simulink model "Longitudinaldynamicmodel_SmartFortwo"  (R2018b)
settings: Solver=FixedStepAuto  StartTime=0.0  StopTime=1  FixedStep=0.01  RelTol=1e-3
values from neighbouring files (symbols this model uses):
  VehMass = 988.5    [Longitudinaldynamicmodel_SmartFortwo_Parameterfile.m]
undefined symbols (not defined in the file or in its folder): DiscIntNeverNeededParam
libraries: Constant_Environment x1, Driver_PI x1, Longitudinal_DrivingCycles x1, Acceleration_Calculation x1, Air_Resistance x1, Roll_Resistance x1, Slope_Resistance x1, Constant_Power_Source x1, Simple_Auxiliary x1, Electric_Drive_Tabled_Consumption x1, Gear_Stage x1, DCAC_Converter x1
(part 2 of 3)

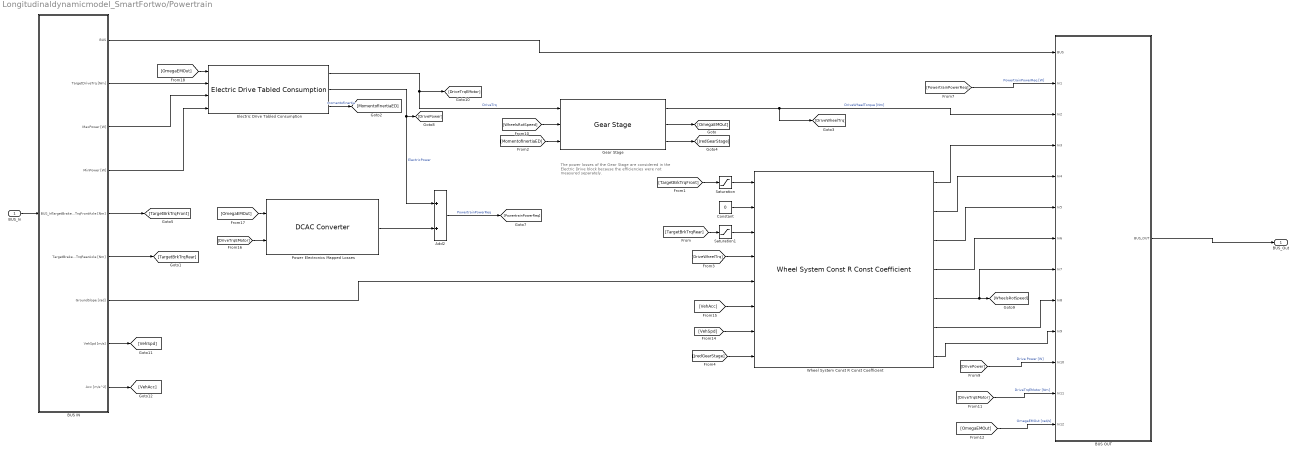
== system Longitudinaldynamicmodel_SmartFortwo/Powertrain ==
  note: The power losses of the Gear Stage are considered
      | in the Electric Drive block because the efficiencies were
      | not measured separately.
  BUS_In : Inport
  Add2 : Sum
  BUS IN : Subsystem
      mask help:
      | <Author> Alexander Koch based on Stefan Müller, Stephan Rohr
      | <Date> 02/05/2017
      |
      | <Description>
      | Automated BUS IN Block for the Bus System. After the Bus In is connected and receives signals it is possible to choose the required signals by clicking on the block. After choosing the signals it is possible to push the Refresh button. This button builds the required amount of outputs, connects the Bus Selector and the Outputs and rename all the outputs with the corresponding signal name.
      |
      | The Block automaticlly disconnects the link to the library block after opening the first time
      |
      | <Parameters>
      | -
      |
      | <Inputs>
      | Bus [Bus]
      |
      | <Outputs>
      | Bus [Bus]
      | SignalName[-]
      mask init:
      | BusInInitFct()
      settings: OpenFcn=|
      | set_param(gcb(),'LinkStatus','none')
      | open_system(gcb(),'mask')
      | open_system(strcat(gcb(),'/Bus Selector'),'Parameter')
      mask DialogControl ParameterGroupVar Prompt: Refresh
      mask DialogControl RefreshOutputs Prompt: Refresh all Output Names
      mask DialogControl RefreshOutputs Callback: BusInInitFct()
  BUS OUT : Subsystem  mask{NumberofInputs=12, NameSys='Powertrain'}
      mask prompts: NumberofInputs "Numper of costum inputs"; NameSys "Name of Bus Subsystem"
      mask help:
      | <Author> Alexander Koch based on Stefan Müller, Stephan Rohr
      | <Date> 02/05/2017
      |
      | <Description>
      | Automated BUS Out Block for the Bus System. Allows to enter the Number of costum inputs and the name of the bus system. After entering the parameters the required amout of Inputs are built and connected to the Bus Creator. The signal names that are connected to the inputs In1, ..., InN are automatically adopted at the Bus signal names and can be found in the Bus under the name of the Bus Subsystem. If the signal (line) to the Inport has no name, the name of the previous blocks outport is taken. If this is not possible, the name if the previous block is taken for the Bus signal name.
      |
      | Additional, there are two buttons. The Refresh Input Names refreshes all Input Names. This is required if signal names are changed or signals are connected for the first time. To build a new system or if another Subsystem is added between existing subsystems, the Refresh Bus Selector is required at every subsystem that is calculated after the new subsystem.
      |
      | The Block automaticlly disconnects the link to the library block after opening the first time
      |
      | <Parameters>
      | Number of costum inputs [-]
      | Name of Bus Subsystem ['abc']
      |
      | <Inputs>
      | Bus [Bus]
      | In1 [ ]
      |
      | <Outputs>
      | Bus [Bus]
      mask init:
      | BusRefreshInputs()
      settings: OpenFcn=|
      | set_param(gcb(),'LinkStatus','none')
      | open_system(gcb(),'mask')
      mask DialogControl Container3 Prompt: Refresh
      mask DialogControl RefreshInputNames Prompt: Refresh Input Names
      mask DialogControl RefreshInputNames Callback: BusRefreshLineNames()
      mask DialogControl RefreshBusSelector Prompt: Refresh Bus Selector
      mask DialogControl RefreshBusSelector Callback: BusRefreshBusSelector()
  Constant : Constant  Value=0
  Electric Drive Tabled Consumption : Electric_Drive_Tabled_Consumption/Electric Drive Tabled Consumption  inertia=0.03  mass=1  OM_M_Pel_Map=[0 84.6925537915840 106.777901162710 132.451481077187 158.717445659769 189.583562564064 219.947567848300 253.359271731562 287.719734913549 325.267898465954 364.560585120281 403.200274983864 447.563591693892 492.828790386663 540.691726349864 590.166785808662 636.561358483905 684.766906055931 734.137596997731 789.985532553104 857.853179816674 908.827398035181 961.684563108046 1019.52904110769 1081.52112973929 1143.57712046773 1200.78427519799 1267.27434692366 1330.96763225908 1399.91145341150 1460.96283186014 1522.13532912128 1591.13337312260 1654.62568484686 1718.49067047593 1783.14030989899 1852.47991946389 1921.56456923299 1990.91312442103 2061.30678608583 2131.34426123832 2203.05270027821 2289.55226312012 2376.68282420177 2454.52733777355 2530.75949498243 2607.34099640618 2684.42711031811 2763.34508226637 2845.97385304829 2963.00280011347 3052.53326845787 3134.40614789669 3225.26823505504 3314.19457665049 3406.50541394017 3500.20227762135 3591.35102796290 3685.03225906601 3782.98250894227 3881.87095410315 3980.79391338854 4076.30627526000 4181.94930220964 4286.97881720375 4389.92406519024 4497.41842284860 4603.47594352982 4710.85061726193 4818.54315585332 4930.22331092001 5041.15761416958 5166.37122862945 5276.81725954101 5387.76544736434 5521.32616802780 5637.26001511646 5761.43879713315 5886.21150930422 6012.17873781274 6142.71364240950 6280.27669163038 5676.19543942961 5258.13958693589 5295.58110214479 5435.21609088646 5171.11785981694 5274.97483494523 5470.31098908416 5158.84365253269 5768.15695867421 5696.91368959506 6048.96408164810 6479.69942526134 6479.69942526134 6479.69942526134 6479.69942526134 6479.69942526134 6479.69942526134 6479.69942526134;0 84.6925537915840 106.777901162710 132.451481077187 158.717445659769 189.583562564064 219.947567848300 253.359271731562 287.719734913549 325.267898465954 364.560585120281 403.200274983864 447.563591693892 492.828790386663 540.691726349864 590.166785808662 636.561358483905 684.766906055931 734.137596997731 789.985532553104 857.853179816674 908.827398035181 961.684563108046 1019.52904110769 1081.52112973929 1143.57712046773 1200.78427519799 1267.27434692366 1330.96763225908 1399.91145341150 1460.96283186014 1522.13532912128 1591.13337312260 1654.62568484686 1718.49067047593 1783.14030989899 1852.47991946389 1921.56456923299 1990.91312442103 2061.30678608583 2131.34426123832 2203.05270027821 2289.55226312012 2376.68282420177 2454.52733777355 2530.75949498243 2607.34099640618 2684.42711031811 2763.34508226637 2845.97385304829 2963.00280011347 3052.53326845787 3134.40614789669 3225.26823505504 3314.19457665049 3406.50541394017 3500.20227762135 3591.35102796290 3685.03225906601 3782.98250894227 3881.87095410315 3980.79391338854 4076.30627526000 4181.94930220964 4286.97881720375 4389.92406519024 4497.41842284860 4603.47594352982 4710.85061726193 4818.54315585332 4930.22331092001 5041.15761416958 5166.37122862945 5276.81725954101 5387.76544736434 5521.32616802780 5637.26001511646 5761.43879713315 5886.21150930422 6012.17873781274 6142.71364240950 6280.27669163038 5676.19543942961 5258.13958693589 5295.58110214479 5435.21609088646 5171.11785981694 5274.97483494523 5470.31098908416 5158.84365253269 5768.15695867421 5696.91368959506 6048.96408164810 6479.69942526134 6479.69942526134 6479.69942526134 6479.69942526134 6479.69942526134 6479.69942526134 6479.69942526134;0 84.6925537915840 106.777901162710 132.451481077187 158.717445659769 189.583562564064 219.947567848300 253.359271731562 287.719734913549 325.267898465954 364.560585120281 403.200274983864 447.563591693892 492.828790386663 540.691726349864 590.166785808662 636.561358483905 684.766906055931 734.137596997731 789.985532553104 857.853179816674 908.827398035181 961.684563108046 1019.52904110769 1081.52112973929 1143.57712046773 1200.78427519799 1267.27434692366 1330.96763225908 1399.91145341150 1460.96283186014 1522.13532912128 1591.13337312260 1654.62568484686 1718.49067047593 1783.14030989899 1852.47991946389 ...(+366716 chars)]  M_MotVector=[0 1.36363636363636 2.72727272727273 4.09090909090909 5.45454545454545 6.81818181818182 8.18181818181818 9.54545454545455 10.9090909090909 12.2727272727273 13.6363636363636 15.0000000000000 16.3636363636364 17.7272727272727 19.0909090909091 20.4545454545455 21.8181818181818 23.1818181818182 24.5454545454545 25.9090909090909 27.2727272727273 28.6363636363636 30.0000000000000 31.3636363636364 32.7272727272727 34.0909090909091 35.4545454545455 36.8181818181818 38.1818181818182 39.5454545454545 40.9090909090909 42.2727272727273 43.6363636363636 45 46.3636363636364 47.7272727272727 49.0909090909091 50.4545454545455 51.8181818181818 53.1818181818182 54.5454545454545 55.9090909090909 57.2727272727273 58.6363636363636 60.0000000000000 61.3636363636364 62.7272727272727 64.0909090909091 65.4545454545455 66.8181818181818 68.1818181818182 69.5454545454546 70.9090909090909 72.2727272727273 73.6363636363636 75 76.3636363636364 77.7272727272727 79.0909090909091 80.4545454545455 81.8181818181818 83.1818181818182 84.5454545454546 85.9090909090909 87.2727272727273 88.6363636363636 90 91.3636363636364 92.7272727272727 94.0909090909091 95.4545454545455 96.8181818181818 98.1818181818182 99.5454545454546 100.909090909091 102.272727272727 103.636363636364 105 106.363636363636 107.727272727273 109.090909090909 110.454545454545 111.818181818182 113.181818181818 114.545454545455 115.909090909091 117.272727272727 118.636363636364 120 121.363636363636 122.727272727273 124.090909090909 125.454545454545 126.818181818182 128.181818181818 129.545454545455 130.909090909091 132.272727272727 133.636363636364 135]  OM_MotVector=[0 3.13202920563366 6.26405841126732 9.39608761690098 12.5281168225346 15.6601460281683 18.7921752338020 21.9242044394356 25.0562336450693 28.1882628507029 31.3202920563366 34.4523212619703 37.5843504676039 40.7163796732376 43.8484088788712 46.9804380845049 50.1124672901386 53.2444964957722 56.3765257014059 59.5085549070395 62.6405841126732 65.7726133183069 68.9046425239405 72.0366717295742 75.1687009352078 78.3007301408415 81.4327593464752 84.5647885521088 87.6968177577425 90.8288469633761 93.9608761690098 97.0929053746435 100.224934580277 103.356963785911 106.488992991544 109.621022197178 112.753051402812 115.885080608445 119.017109814079 122.149139019713 125.281168225346 128.413197430980 131.545226636614 134.677255842247 137.809285047881 140.941314253515 144.073343459148 147.205372664782 150.337401870416 153.469431076049 156.601460281683 159.733489487317 162.865518692950 165.997547898584 169.129577104218 172.261606309851 175.393635515485 178.525664721119 181.657693926752 184.789723132386 187.921752338020 191.053781543653 194.185810749287 197.317839954921 200.449869160554 203.581898366188 206.713927571822 209.845956777455 212.977985983089 216.110015188723 219.242044394356 222.374073599990 225.506102805624 228.638132011257 231.770161216891 234.902190422524 238.034219628158 241.166248833792 244.298278039425 247.430307245059 250.562336450693 253.694365656326 256.826394861960 259.958424067594 263.090453273227 266.222482478861 269.354511684495 272.486540890128 275.618570095762 278.750599301396 281.882628507029 285.014657712663 288.146686918297 291.278716123930 294.410745329564 297.542774535198 300.674803740831 303.806832946465 306.938862152099 310.070891357732 313.202920563366 316.334949769000 319.466978974633 322.599008180267 325.731037385901 328.863066591534 331.995095797168 335.127125002802 338.259154208435 341.391183414069 344.523212619703 347.655241825336 350.787271030970 353.919300236604 357.051329442237 360.183358647871 363.315387853505 366.447417059138 369.579446264772 372.711475470406 375.843504676039 378.975533881673 382.107563087307 385.239592292940 388.371621498574 391.503650704208 394.635679909841 397.767709115475 400.899738321108 404.031767526742 407.163796732376 410.295825938009 413.427855143643 416.559884349277 419.691913554910 422.823942760544 425.955971966178 429.088001171811 432.220030377445 435.352059583079 438.484088788712 441.616117994346 444.748147199980 447.880176405613 451.012205611247 454.144234816881 457.276264022514 460.408293228148 463.540322433782 466.672351639415 469.804380845049 472.936410050683 476.068439256316 479.200468461950 482.332497667584 485.464526873217 488.596556078851 491.728585284485 494.860614490118 497.992643695752 501.124672901386 504.256702107019 507.388731312653 510.520760518287 513.652789723920 516.784818929554 519.916848135188 523.048877340821 526.180906546455 529.312935752089 532.444964957722 535.576994163356 538.709023368990 541.841052574623 544.973081780257 548.105110985890 551.237140191524 554.369169397158 557.501198602791 560.633227808425 563.765257014059 566.897286219692 570.029315425326 573.161344630960 576.293373836593 579.425403042227 582.557432247861 585.689461453494 588.821490659128 591.953519864762 595.085549070395 598.217578276029 601.349607481663 604.481636687296 607.613665892930 610.745695098564 613.877724304197 617.009753509831 620.141782715465 623.273811921098 626.405841126732 629.537870332366 632.669899537999 635.801928743633 638.933957949267 642.065987154900 645.198016360534 648.330045566168 651.462074771801 654.594103977435 657.726133183069 660.858162388702 663.990191594336 667.122220799970 670.254250005603 673.386279211237 676.518308416871 679.650337622504 682.782366828138 685.914396033772]  M_Full_Load=[128 128 128 127 127 126 126 126 126 124 119 114 109 103 100 94 89 85 79 75 70 68 67 65 63 62 60 58 59 60 62 63 63 62 61 60 58 57 55 53 51 50 48 46 45 43 42 40 39 38 36 35 34 32 31 30 29 28 26 25 24]  OM_Full_Load=[0 11.4144533080429 22.8289066160858 34.2433599241288 45.6578132321717 57.1769862953342 68.5914396033771 80.0058929114201 91.4203462194630 102.834799527506 114.249252835549 125.663706143592 137.078159451635 148.492612759678 160.011785822840 171.426239130883 182.840692438926 194.255145746969 205.669599055012 217.084052363055 228.498505671098 239.912958979141 251.327412287183 262.846585350346 274.261038658389 285.675491966432 297.089945274475 308.504398582518 319.918851890561 331.333305198604 342.747758506646 354.162211814689 365.681384877852 377.095838185895 388.510291493938 399.924744801981 411.339198110024 422.753651418066 434.168104726109 445.582558034152 456.997011342195 468.516184405358 479.930637713401 491.345091021444 502.759544329487 514.173997637529 525.588450945572 537.002904253615 548.417357561658 559.831810869701 571.350983932864 582.765437240907 594.179890548950 605.594343856992 617.008797165035 628.423250473078 639.837703781121 651.252157089164 662.666610397207 674.185783460370 685.600236768413]  M_Min_Load=[0 0 0 0 0 0 0 0 0 0 0 0 0 0 0 0 0 0 0 0 0 0 0 0 0 0 0 0 0 0 0 0 0 0 0 0 0 0 0 0 0 0 0 0 0 0 0 0 0 0 0 0 0 0 0 0 0 0 0 0 0]  OM_Min_Load=[0 11.4144533080429 22.8289066160858 34.2433599241288 45.6578132321717 57.1769862953342 68.5914396033771 80.0058929114201 91.4203462194630 102.834799527506 114.249252835549 125.663706143592 137.078159451635 148.492612759678 160.011785822840 171.426239130883 182.840692438926 194.255145746969 205.669599055012 217.084052363055 228.498505671098 239.912958979141 251.327412287183 262.846585350346 274.261038658389 285.675491966432 297.089945274475 308.504398582518 319.918851890561 331.333305198604 342.747758506646 354.162211814689 365.681384877852 377.095838185895 388.510291493938 399.924744801981 411.339198110024 422.753651418066 434.168104726109 445.582558034152 456.997011342195 468.516184405358 479.930637713401 491.345091021444 502.759544329487 514.173997637529 525.588450945572 537.002904253615 548.417357561658 559.831810869701 571.350983932864 582.765437240907 594.179890548950 605.594343856992 617.008797165035 628.423250473078 639.837703781121 651.252157089164 662.666610397207 674.185783460370 685.600236768413]  LocalSampleTime=-1
  Gear Stage : Gear_Stage/Gear Stage  iGear=i_gear  eta=1  JredGetr=0.19  LocalSampleTime=-1
  Power Electronics Mapped Losses : DCAC_Converter/DCAC Converter  W_Vektor=[0 10.4719755119660 21.7817090648892 33.0914426178125 44.4011761707357 55.7109097236590 67.0206432765823 78.3303768295055 89.6401103824288 100.949843935352 112.259577488275 123.569311041199 134.879044594122 146.188778147045 157.498511699968 168.808245252892 180.117978805815 191.427712358738 202.737445911661 214.047179464585 225.356913017508 236.666646570431 247.976380123354 259.286113676278 270.595847229201 281.905580782124 293.215314335047 304.525047887971 315.834781440894 327.144514993817 338.454248546740 349.763982099664 361.073715652587 372.383449205510 383.693182758433 395.002916311357 406.312649864280 417.622383417203 428.932116970126 440.241850523050 451.551584075973 462.861317628896 474.171051181819 485.480784734743 496.790518287666 508.100251840589 519.409985393512 530.719718946436 542.029452499359 553.339186052282 564.648919605206 575.958653158129 587.268386711052 598.578120263975 609.887853816898 621.197587369822 632.507320922745 643.817054475668 655.126788028592 666.436521581515 677.746255134438]  M_Vektor_motgen=[0 1 2 3 4 5 6 7 8 9 10 11 12 13 14 15 16 17 18 19 20 21 22 23 24 25 26 27 28 29 30 31 32 33 34 35 36 37 38 39 40 41 42 43 44 45 46 47 48 49 50 51 52 53 54 55 56 57 58 59 60 61 62 63 64 65 66 67 68 69 70 71 72 73 74 75 76 77 78 79 80 81 82 83 84 85 86 87 88 89 90 91 92 93 94 95 96 97 98 99 100 101 102 103 104 105 106 107 108 109 110 111 112 113 114 115 116 117 118 119 120 121 122 123 124 125 126 127 128 129 130]  P_Loss=[0 0 0 0 0 0 0 0 0 0 0 0 0 0 0 0 0 0 0 0 0 0 0 0 0 0 0 0 0 0 0 0 0 0 0 0 0 0 0 0 0 0 0 0 0 0 0 0 0 0 0 0 0 0 0 0 0 0 0 0 0 0 0 0 0 0 0 0 0 0 0 0 0 0 0 0 0 0 0 0 0 0 0 0 0 0 0 0 0 0 0 0 0 0 0 0 0 0 0 0 0 0 0 0 0 0 0 0 0 0 0 0 0 0 0 0 0 0 0 0 0 0 0 0 0 0 0 0 0 0 0;0 82 70 84 90 100 106 112 101 115 122 130 144 146 153 162 154 169 188 198 202 216 231 236 247 260 271 279 293 309 316 326 335 353 373 392 407 427 437 460 475 478 493 505 523 529 551 565 570 582 598 616 631 647 665 682 700 716 730 726 743 763 780 805 824 840 861 884 903 919 947 960 981 995 1018 1041 1062 1086 1110 1130 1152 1170 1188 1211 1237 1259 1280 1302 1323 1344 1369 1392 1412 1440 1460 1493 1518 1540 1568 1594 1617 1646 1670 1709 1743 1769 1791 1825 1856 1881 1938 2212 3001 3444 3441 3510 3626 3825 3876 3879 3957 4140 4177 3954 4094 3971 3839 3839 3839 3839 3839;0 61 78 75 74 73 81 94 94 97 96 106 120 131 139 145 154 169 180 188 198 206 215 230 242 254 265 268 286 302 306 318 344 370 384 399 410 423 438 458 483 500 512 520 528 539 554 573 589 600 614 632 645 655 678 691 714 720 739 748 763 777 787 809 833 829 860 887 913 937 949 962 976 988 1007 1032 1049 1076 1095 1118 1143 1168 1192 1212 1231 1256 1293 1323 1337 1356 1387 1406 1427 1456 1469 1496 1515 1558 1577 1607 1643 1675 1694 1710 1739 1772 1805 1832 1870 1893 1924 1942 1976 1999 2049 2640 3767 4034 4108 4084 4241 4351 4407 4486 4544 4620 3839 3839 3839 3839 3839;0 70 71 95 83 94 92 96 105 107 112 125 141 143 150 153 165 176 190 203 218 233 240 245 253 260 274 285 304 329 341 352 358 365 379 403 424 444 460 472 483 499 525 535 543 561 575 589 597 611 632 643 656 664 677 700 719 731 742 759 777 794 814 839 858 870 892 917 938 953 968 987 1008 1022 1035 1055 1085 1111 1129 1151 1176 1192 1213 1240 1276 1296 1325 1348 1369 1387 1405 1432 1465 1493 1507 1525 1558 1586 1614 1642 1663 1683 1718 1753 1777 1801 1832 1860 1893 1925 1956 1984 2007 2030 2062 2093 2124 2160 2187 2222 2252 2304 2714 4353 4916 3997 3839 3839 3839 3839 3839;0 74 50 130 190 192 101 114 128 71 125 147 164 97 157 185 186 201 216 227 232 238 241 252 264 279 293 306 320 335 355 350 365 394 396 405 423 436 452 468 481 497 508 518 532 545 554 569 588 604 613 625 645 667 677 690 709 726 745 765 780 791 803 829 843 855 881 897 912 926 942 967 994 1017 1036 1056 1073 1104 1121 1152 1181 1210 1240 1264 1282 1303 1323 1349 1371 1396 1415 1439 1469 1495 1515 1540 1563 1591 1625 1648 1677 1706 1736 1764 1793 1824 1842 1877 1912 1945 1975 2002 2024 2048 2081 2116 2143 2180 2207 2259 2278 2340 2348 2402 2412 3130 3839 3839 3839 3839 3839;0 97 63 80 77 71 70 92 102 101 123 143 135 155 167 123 148 166 185 200 226 242 265 255 265 280 315 323 318 335 346 366 381 399 417 422 439 455 469 485 498 512 525 539 550 574 587 589 608 620 642 662 668 685 705 718 725 738 758 776 792 805 834 852 859 885 897 923 947 967 985 998 1012 1023 1052 1079 1100 1125 1143 1167 1187 1214 1253 1276 1309 1333 1360 1375 1400 1424 1445 1464 1482 1504 1536 1562 1591 1615 1648 1680 1708 1734 1763 1796 1819 1825 1852 1870 1910 1946 1979 2013 2048 2088 2118 2153 2189 2216 2239 2276 2311 2337 2377 2430 2439 3130 3839 3839 3839 3839 3839;0 54 47 58 68 60 51 67 76 84 98 114 113 116 128 138 140 157 175 171 180 195 214 221 231 239 258 265 274 290 315 334 355 377 405 415 432 449 467 482 502 518 521 532 552 558 572 584 600 622 634 651 666 679 694 714 726 740 762 782 800 820 833 853 876 894 914 931 953 971 981 991 1011 1036 1068 1088 1111 1128 1142 1166 1197 1229 1255 1273 1304 1348 1379 1414 1440 1454 1475 1496 1514 1537 1564 1589 1611 1605 1652 1678 1706 1735 1768 1805 1835 1862 1903 1936 1962 2002 2036 2057 2079 2113 2149 2183 2212 2244 2285 2323 2355 2386 2410 2437 2457 3130 3839 3839 3839 3839 3839;0 78 78 96 96 93 93 106 115 120 127 134 146 157 157 161 179 196 182 188 211 212 224 245 260 287 306 309 317 325 338 356 376 399 405 416 447 470 487 494 492 494 517 534 542 561 575 584 604 625 635 656 668 681 703 723 742 765 786 804 816 829 843 864 889 904 916 929 942 962 992 1019 1036 1061 1082 ...(+31348 chars)]  LocalSampleTime=-1
  Saturation : Saturate  UpperLimit=0  LowerLimit=-inf
  Saturation1 : Saturate  UpperLimit=0  LowerLimit=-inf
  Wheel System Const R Const Coefficient : Wheel_System_Const_R/Wheel System Const R Const Coefficient  Wheel_Radius=r_dyn  Wheel_Roll_Resistance=0.0185  Wheel_Roll_Resistance_Dyn=0  mu_Tyre=0.7  J_FourWheels=4  Gravity=gravity  Wheelbase=1.863  COG_Height=0.5  COG_Front=1.1178  COG_Rear=0.7452  Veh_Mass=VehMass  LocalSampleTime=-1
  BUS_Out : Outport
  wires:
  BUS IN/1(BUS) -> BUS OUT/1(BUS)
  BUS_In/1 -> BUS IN/1(BUS_In)
  [TargetBrkTrqFront] -> Saturation/1
  [TargetBrkTrqRear] -> Saturation1/1
  BUS IN/5(TargetBrakeTrqFrontAxle [Nm]) -> [TargetBrkTrqFront]
  BUS IN/2(TargetDriveTrq [Nm]) -> Electric Drive Tabled Consumption/2
  Electric Drive Tabled Consumption/1 -> Gear Stage/1, [DriveTrqEMotor]  "DriveTrq"
  Gear Stage/2 -> [OmegaEMOut]
  Constant/1 -> Wheel System Const R Const Coefficient/2
  [MomentofInertiaED] -> Gear Stage/3
  Gear Stage/1 -> [DriveWheelTrq], BUS OUT/3(In2)  "DriveWheelTorque [Nm]"
  [DriveWheelTrq] -> Wheel System Const R Const Coefficient/4
  Gear Stage/3 -> [JredGearStage]
  [JredGearStage] -> Wheel System Const R Const Coefficient/8
  Wheel System Const R Const Coefficient/1 -> BUS OUT/4(In3)
  Wheel System Const R Const Coefficient/2 -> BUS OUT/5(In4)
  Wheel System Const R Const Coefficient/3 -> BUS OUT/6(In5)
  Wheel System Const R Const Coefficient/4 -> BUS OUT/7(In6)
  Wheel System Const R Const Coefficient/5 -> [WheelsRotSpeed], BUS OUT/8(In7)
  Wheel System Const R Const Coefficient/6 -> BUS OUT/9(In8)
  Wheel System Const R Const Coefficient/7 -> BUS OUT/10(In9)
  Electric Drive Tabled Consumption/2 -> Add2/1, [DrivePower]  "ElectricPower"
  Add2/1 -> [PowertrainPowerReq]  "PowertrainPowerReq"
  BUS IN/7(GroundSlope [rad]) -> Wheel System Const R Const Coefficient/5
  Saturation/1 -> Wheel System Const R Const Coefficient/1
  Saturation1/1 -> Wheel System Const R Const Coefficient/3
  [PowertrainPowerReq] -> BUS OUT/2(In1)  "PowertrainPowerReq [W]"
  [DrivePower] -> BUS OUT/11(In10)  "Drive Power [W]"
  [WheelsRotSpeed] -> Gear Stage/2
  [DriveTrqEMotor] -> BUS OUT/12(In11)  "DriveTrqEMotor [Nm]"
  [OmegaEMOut] -> BUS OUT/13(In12)  "OmegaEMOut [rad/s]"
  BUS IN/6(TargetBrakeTrqRearAxle [Nm]) -> [TargetBrkTrqRear]
  BUS IN/8(VehSpd [m/s]) -> [VehSpd]
  [VehSpd] -> Wheel System Const R Const Coefficient/7
  BUS IN/9(Acc [m/s^2]) -> [VehAcc]
  [VehAcc] -> Wheel System Const R Const Coefficient/6
  [DriveTrqEMotor] -> Power Electronics Mapped Losses/2
  [OmegaEMOut] -> Power Electronics Mapped Losses/1
  Power Electronics Mapped Losses/1 -> Add2/2
  [OmegaEMOut] -> Electric Drive Tabled Consumption/1
  Electric Drive Tabled Consumption/3 -> [MomentofInertiaED]  "momentofinertia"
  BUS IN/3(MaxPower [W]) -> Electric Drive Tabled Consumption/3
  BUS IN/4(MinPower [W]) -> Electric Drive Tabled Consumption/4
  BUS OUT/1(BUS_OUT) -> BUS_Out/1
